simulink model "sst"  (R2025a)
settings: Solver=ode1be  StartTime=0.0  StopTime=simlength  FixedStep=tc  MaxStep=ts_sim
values from neighbouring files (symbols this model uses):
  Adrso = eye(2) + Arso*ts_inv    [design_model.m]
  alpha = 35    [design_model.m]
  C1 = 0.5    [design_model.m]
  Crso = [1 0]    [design_model.m]
  DThs_init = 0    [design_model.m]
  E0 = 3.485    [design_model.m]
  E1 = 0.2156    [design_model.m]
  E2 = 0    [design_model.m]
  E3 = 0    [design_model.m]
  E_1 = -1.031    [design_model.m]
  Elog = -0.05    [design_model.m]
  fPWM_DAB = fPWM_INV    (= 35000)    [design_model.m]
  fPWM_INV = 35e3    (= 35000)    [design_model.m]
  freq = 50    [design_model.m]
  I_FS = Iout_ac_rms_nom * sqrt(2) * margin_factor    [design_model.m]
  ki_i_dab = 18    [design_model.m]
  ki_pll = 3140    [design_model.m]
  ki_v_dab = 45    [design_model.m]
  kp_i_dab = 2    [design_model.m]
  kp_pll = 314    [design_model.m]
  kp_v_dab = 8    [design_model.m]
  Ldrso = acker(Adrso',Crso',polesdrso)'    [design_model.m]
  M = 125    [design_model.m]
  number_of_cells = 30    [design_model.m]
  Q = 1000    [design_model.m]
  q1Kalman = ts_inv^2    (= 8.16326530612e-10)    [design_model.m]
  q2Kalman = ts_inv^1    (= 2.85714285714e-05)    [design_model.m]
  q3Kalman = 0    [design_model.m]
  R0 = 0.0035    [design_model.m]
  R1 = 0.0035    [design_model.m]
  rKalman = 1    [design_model.m]
  Tambient = 40    [design_model.m]
  tc = ts_inv/200    (= 1.42857142857e-07)    [design_model.m]
  ts_afe = ts_inv    (= 2.85714285714e-05)    [design_model.m]
  ts_dab = tPWM_DAB*2    (= 5.71428571429e-05)    [design_model.m]
  ts_inv = tPWM_INV    (= 2.85714285714e-05)    [design_model.m]
  V_FS = Vout_dc_nom * margin_factor    (= 500)    [design_model.m]
  weigth = 0.6/6    (= 0.1)    [design_model.m]
undefined symbols (not defined in the file or in its folder): Aresd, Bresd, Cresd, dead_time_DAB, dead_time_INV, iph_grid_pu_ref, ki_afe, kp_afe, LFu1_AFE, n_modules, omega_grid_nom, RLFu1_AFE, ts_battery, tsample, V_phase_normalization_factor, Vdab2_dc_nom
libraries: fl_lib x280, nesl_utility x188, ee_lib x41, cstblocks x4, single_phase_transformer_lib x2, lithium_ion_cell_lib x1, simulink x1
(part 2 of 12)

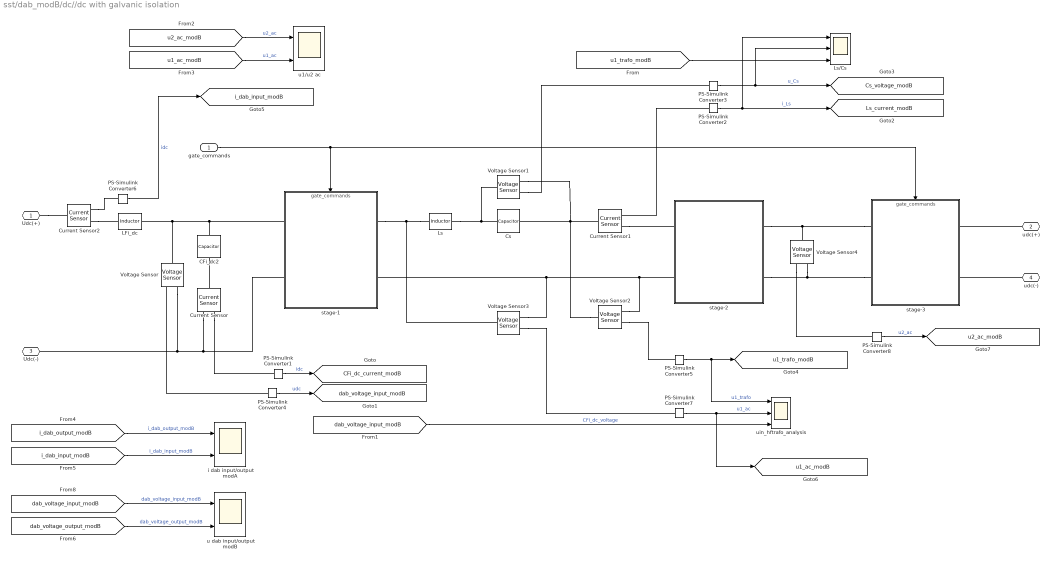
== system sst/dab_modB/dc//dc with galvanic isolation ==
  gate_commands : Inport
  CFi_dc2 : fl_lib/Electrical/Electrical Elements/Capacitor  c=CFi_dc1 F  r=RCFi_dc1_internal Ohm  g=0 1/Ohm  i_specify=off  i_priority=None  i=0 A  i_nominal_specify=off  i_nominal_value=1  i_nominal_unit=A  v_specify=off  v_priority=None  v=0 V  v_nominal_specify=off  v_nominal_value=1  v_nominal_unit=V  vc_specify=off  vc_priority=High  vc=0 V  vc_nominal_specify=off  vc_nominal_value=1  vc_nominal_unit=V
  Cs : fl_lib/Electrical/Electrical Elements/Capacitor  c=Cs1 F  r=1e-6 Ohm  g=0 1/Ohm  i_specify=off  i_priority=None  i=0 A  i_nominal_specify=off  i_nominal_value=1  i_nominal_unit=A  v_specify=off  v_priority=None  v=0 V  v_nominal_specify=off  v_nominal_value=1  v_nominal_unit=V  vc_specify=off  vc_priority=High  vc=0 V  vc_nominal_specify=off  vc_nominal_value=1  vc_nominal_unit=V
  Current Sensor : fl_lib/Electrical/Electrical Sensors/Current Sensor
  Current Sensor1 : fl_lib/Electrical/Electrical Sensors/Current Sensor
  Current Sensor2 : fl_lib/Electrical/Electrical Sensors/Current Sensor
  LFi_dc : fl_lib/Electrical/Electrical Elements/Inductor  l=LFi_dc H  r=RLFi_dc Ohm  g=1e-9 1/Ohm  i_specify=off  i_priority=None  i=0 A  i_nominal_specify=off  i_nominal_value=1  i_nominal_unit=A  v_specify=off  v_priority=None  v=0 V  v_nominal_specify=off  v_nominal_value=1  v_nominal_unit=V  i_L_specify=off  i_L_priority=High  i_L=0 A  i_L_nominal_specify=off  i_L_nominal_value=1  i_L_nominal_unit=A
  Ls : fl_lib/Electrical/Electrical Elements/Inductor  l=Ls1 H  r=0 Ohm  g=1e-9 1/Ohm  i_specify=off  i_priority=None  i=0 A  i_nominal_specify=off  i_nominal_value=1  i_nominal_unit=A  v_specify=off  v_priority=None  v=0 V  v_nominal_specify=off  v_nominal_value=1  v_nominal_unit=V  i_L_specify=off  i_L_priority=High  i_L=0 A  i_L_nominal_specify=off  i_L_nominal_value=1  i_L_nominal_unit=A
  Ls/Cs : Scope  NumInputPorts=3
      settings: SampleTime=tc  ActiveDisplayYMinimum=-8555.3769671330647  ActiveDisplayYMaximum=8509.2940450823044
  PS-Simulink Converter1 : nesl_utility/PS-Simulink Converter  PhysicalDomain=network_engine_domain  SubClassName=ps_output  LeftPortType=input  RightPortType=output  PseudoPeriodic=off  Frequencies=[]  VectorFormat=1-D array  Unit=A  AffineConversion=on
  PS-Simulink Converter2 : nesl_utility/PS-Simulink Converter  PhysicalDomain=network_engine_domain  SubClassName=ps_output  LeftPortType=input  RightPortType=output  PseudoPeriodic=off  Frequencies=[]  VectorFormat=1-D array  Unit=A  AffineConversion=on
  PS-Simulink Converter{3..5,7..8} (5 alike) : nesl_utility/PS-Simulink Converter  PhysicalDomain=network_engine_domain  SubClassName=ps_output  LeftPortType=input  RightPortType=output  PseudoPeriodic=off  Frequencies=[]  VectorFormat=1-D array  Unit=V  AffineConversion=on
  PS-Simulink Converter6 : nesl_utility/PS-Simulink Converter  PhysicalDomain=network_engine_domain  SubClassName=ps_output  LeftPortType=input  RightPortType=output  PseudoPeriodic=off  Frequencies=[]  VectorFormat=1-D array  Unit=A  AffineConversion=on
  Voltage Sensor{,1..4} (5 alike) : fl_lib/Electrical/Electrical Sensors/Voltage Sensor
  i dab input/output modA : Scope  NumInputPorts=2
      settings: SampleTime=tc  ActiveDisplayYMinimum=49.856547808264907  ActiveDisplayYMaximum=125.72881684551226  DataLoggingVariableName=ScopeData9
  stage-1 : Subsystem
      settings: PortSchema="{\"entries\":[{\"content\":{\"sides\":[{\"content\":{\"connectorIds\":[\"LConn1\",\"LConn2\"]},\"type\":\"ConnectorPlacement.EquallySpacedRectSide\",\"uuid\":\"c872503a-61af-4937-bdf2-4de4f8645573\"},{\"content\":{\"connectorIds\":[\"RConn1\",\"RConn2\"],\"side\":\"RIGHT\"},\"type\":\"ConnectorPlacement.EquallySpacedRectSide\",\"uuid\":\"3b83f060-86a2-4569-84b5-d9f7c0485347\"},{\"content\":{\"connectorIds\":[\"In1\"],\"side\":\"TOP\"},\"type\":\"ConnectorPlacement.EquallySpacedRectSide\",\"uuid\":\"bf191d46-ce71-4d15-9dd0-24cc57253577\"}]},\"type\":\"ConnectorPlacement.EquallySpacedConnector\",\"uuid\":\"1b28ceee-25d0-45ae-a3c4-c2563f0d63ba\"}],\"packageUris\":[\"http://schema.mathworks.com/mf0/Connector/R2020b\"],\"version\":\"1.0\"}"
  stage-2 : Subsystem
  stage-3 : Subsystem
      settings: PortSchema="{\"entries\":[{\"content\":{\"sides\":[{\"content\":{\"connectorIds\":[\"LConn1\",\"LConn2\"]},\"type\":\"ConnectorPlacement.EquallySpacedRectSide\",\"uuid\":\"c872503a-61af-4937-bdf2-4de4f8645573\"},{\"content\":{\"connectorIds\":[\"RConn1\",\"RConn2\"],\"side\":\"RIGHT\"},\"type\":\"ConnectorPlacement.EquallySpacedRectSide\",\"uuid\":\"3b83f060-86a2-4569-84b5-d9f7c0485347\"},{\"content\":{\"connectorIds\":[\"In1\"],\"side\":\"TOP\"},\"type\":\"ConnectorPlacement.EquallySpacedRectSide\",\"uuid\":\"bf191d46-ce71-4d15-9dd0-24cc57253577\"}]},\"type\":\"ConnectorPlacement.EquallySpacedConnector\",\"uuid\":\"1b28ceee-25d0-45ae-a3c4-c2563f0d63ba\"}],\"packageUris\":[\"http://schema.mathworks.com/mf0/Connector/R2020b\"],\"version\":\"1.0\"}"
  u dab input/output modB : Scope  NumInputPorts=2
      settings: SampleTime=tc  ActiveDisplayYMinimum=-3745.5802333321844  ActiveDisplayYMaximum=2860.9744612967625  DataLoggingVariableName=ScopeData11
  u1/u2 ac : Scope  NumInputPorts=2
      settings: SampleTime=tc  ActiveDisplayYMinimum=-24024.630641506188  ActiveDisplayYMaximum=24011.441993829012  DataLoggingVariableName=ScopeData5
  uin_hftrafo_analysis : Scope  NumInputPorts=3
      settings: SampleTime=tc  ActiveDisplayYMinimum=-13105.49054417162  ActiveDisplayYMaximum=11952.045335245366
  Udc(+) : PMIOPort  Side=Left
  udc(+) : PMIOPort  Port=2  Side=Right
  Udc(-) : PMIOPort  Port=3  Side=Left
  udc(-) : PMIOPort  Port=4  Side=Right
  tag scope: CFi_dc_current_modB=global, Cs_voltage_modB=global, Ls_current_modB=global, dab_voltage_input_modB=global, i_dab_input_modB=global, u1_ac_modB=global, u1_trafo_modB=global, u2_ac_modB=global
  wires:
  [u1_ac_modB] -> u1/u2 ac/2  "u1_ac"
  [u2_ac_modB] -> u1/u2 ac/1  "u2_ac"
  PS-Simulink Converter8/1 -> [u2_ac_modB]  "u2_ac"
  PS-Simulink Converter6/1 -> [i_dab_input_modB]  "idc"
  [dab_voltage_input_modB] -> uin_hftrafo_analysis/3  "CFi_dc_voltage"
  PS-Simulink Converter7/1 -> uin_hftrafo_analysis/2, [u1_ac_modB]  "u1_ac"
  [u1_trafo_modB] -> Ls/Cs/3
  PS-Simulink Converter5/1 -> [u1_trafo_modB], uin_hftrafo_analysis/1  "u1_trafo"
  PS-Simulink Converter3/1 -> [Cs_voltage_modB], Ls/Cs/2  "u_Cs"
  PS-Simulink Converter2/1 -> [Ls_current_modB], Ls/Cs/1  "i_Ls"
  PS-Simulink Converter4/1 -> [dab_voltage_input_modB]  "udc"
  PS-Simulink Converter1/1 -> [CFi_dc_current_modB]  "idc"
  gate_commands/1 -> stage-1/1(gate_commands), stage-3/1(gate_commands)
  [i_dab_input_modB] -> i dab input/output modA/2  "i_dab_input_modB"
  [i_dab_output_modB] -> i dab input/output modA/1  "i_dab_output_modB"
  [dab_voltage_input_modB] -> u dab input/output modB/1  "dab_voltage_input_modB"
  [dab_voltage_output_modB] -> u dab input/output modB/2  "dab_voltage_output_modB"
  connections:
  Voltage Sensor4/RConn1 -- PS-Simulink Converter8/LConn1
  Current Sensor2/RConn1 -- PS-Simulink Converter6/LConn1
  Udc(+)/RConn1 -- Current Sensor2/LConn1
  Current Sensor2/RConn2 -- LFi_dc/LConn1
  udc(-)/RConn1 -- stage-3/RConn2
  udc(+)/RConn1 -- stage-3/RConn1
  stage-3/LConn2 -- Voltage Sensor4/RConn2 -- stage-2/RConn2
  stage-3/LConn1 -- Voltage Sensor4/LConn1 -- stage-2/RConn1
  Voltage Sensor3/RConn1 -- PS-Simulink Converter7/LConn1
  Voltage Sensor1/LConn1 -- Cs/LConn1 -- Ls/RConn1
  Voltage Sensor2/LConn1 -- Cs/RConn1 -- Current Sensor1/LConn1 -- Voltage Sensor1/RConn2
  Voltage Sensor2/RConn1 -- PS-Simulink Converter5/LConn1
  Voltage Sensor1/RConn1 -- PS-Simulink Converter3/LConn1
  PS-Simulink Converter2/LConn1 -- Current Sensor1/RConn1
  Current Sensor1/RConn2 -- stage-2/LConn1
  Ls/LConn1 -- Voltage Sensor3/LConn1 -- stage-1/LConn1
  PS-Simulink Converter4/LConn1 -- Voltage Sensor/RConn1
  Current Sensor/RConn1 -- PS-Simulink Converter1/LConn1
  Current Sensor/LConn1 -- CFi_dc2/RConn1
  Voltage Sensor/RConn2 -- Udc(-)/RConn1 -- Current Sensor/RConn2 -- stage-1/RConn2
  Voltage Sensor/LConn1 -- LFi_dc/RConn1 -- CFi_dc2/LConn1 -- stage-1/RConn1
  Voltage Sensor3/RConn2 -- stage-1/LConn2 -- Voltage Sensor2/RConn2 -- stage-2/LConn2

== system sst/dab_modB/single_phase_ui_measure1 ==
  Bus Creator : BusCreator  Inputs=2
  Current Sensor : fl_lib/Electrical/Electrical Sensors/Current Sensor
  Selector : Selector  InputPortWidth=2  IndexOptions=Index vector (dialog)  Indices=2  OutputSizes=1
  Selector1 : Selector  InputPortWidth=2  IndexOptions=Index vector (dialog)  Indices=1  OutputSizes=1
  Voltage Sensor : fl_lib/Electrical/Electrical Sensors/Voltage Sensor
  dab input modB : Scope  NumInputPorts=2
      settings: SampleTime=tc  ActiveDisplayYMinimum=-212.36678678828113  ActiveDisplayYMaximum=307.17150645761535  DataLoggingVariableName=ScopeData2
  iph : nesl_utility/PS-Simulink Converter  PhysicalDomain=network_engine_domain  SubClassName=ps_output  LeftPortType=input  RightPortType=output  PseudoPeriodic=off  Frequencies=[]  VectorFormat=1-D array  Unit=A  AffineConversion=off
  uph : nesl_utility/PS-Simulink Converter  PhysicalDomain=network_engine_domain  SubClassName=ps_output  LeftPortType=input  RightPortType=output  PseudoPeriodic=off  Frequencies=[]  VectorFormat=1-D array  Unit=V  AffineConversion=off
  Udc(+) : PMIOPort  Side=Left
  udc(+) : PMIOPort  Port=2  Side=Right
  Udc(-) : PMIOPort  Port=3  Side=Left
  udc(-) : PMIOPort  Port=4  Side=Right
  tag scope: current_battery_modB=global, voltage_battery_modB=global
  wires:
  Selector/1 -> [voltage_battery_modB], dab input modB/2  "voltage_battery"
  Selector1/1 -> dab input modB/1, [current_battery_modB]  "current_battery"
  uph/1 -> Bus Creator/2  "uph"
  iph/1 -> Bus Creator/1  "iph"
  Bus Creator/1 -> Selector1/1, Selector/1  "ui_data"
  connections:
  udc(-)/RConn1 -- Udc(-)/RConn1 -- Voltage Sensor/RConn2
  Voltage Sensor/RConn1 -- uph/LConn1
  Current Sensor/RConn2 -- udc(+)/RConn1
  Udc(+)/RConn1 -- Current Sensor/LConn1 -- Voltage Sensor/LConn1
  iph/LConn1 -- Current Sensor/RConn1

== system sst/dab_modB/ui_measure ==
  Bus Creator : BusCreator  Inputs=2
  Current Sensor : fl_lib/Electrical/Electrical Sensors/Current Sensor
  Selector : Selector  InputPortWidth=2  IndexOptions=Index vector (dialog)  Indices=2  OutputSizes=1
  Selector1 : Selector  InputPortWidth=2  IndexOptions=Index vector (dialog)  Indices=1  OutputSizes=1
  Voltage Sensor : fl_lib/Electrical/Electrical Sensors/Voltage Sensor
  dab output modB : Scope  NumInputPorts=2
      settings: SampleTime=tc  ActiveDisplayYMinimum=-324379.544123381  ActiveDisplayYMaximum=2.4176410117358118E+6  DataLoggingVariableName=ScopeData2
  iph : nesl_utility/PS-Simulink Converter  PhysicalDomain=network_engine_domain  SubClassName=ps_output  LeftPortType=input  RightPortType=output  PseudoPeriodic=off  Frequencies=[]  VectorFormat=1-D array  Unit=A  AffineConversion=off
  uph : nesl_utility/PS-Simulink Converter  PhysicalDomain=network_engine_domain  SubClassName=ps_output  LeftPortType=input  RightPortType=output  PseudoPeriodic=off  Frequencies=[]  VectorFormat=1-D array  Unit=V  AffineConversion=off
  Udc(+) : PMIOPort  Side=Left
  udc(+) : PMIOPort  Port=2  Side=Right
  Udc(-) : PMIOPort  Port=3  Side=Left
  udc(-) : PMIOPort  Port=4  Side=Right
  tag scope: dab_current_output_modB=global, dab_voltage_output_modB=global
  wires:
  uph/1 -> Bus Creator/2  "uph"
  iph/1 -> Bus Creator/1  "iph"
  Bus Creator/1 -> Selector1/1, Selector/1  "ui_data"
  Selector/1 -> [dab_voltage_output_modB]
  Selector1/1 -> [dab_current_output_modB]
  [dab_voltage_output_modB] -> dab output modB/2  "dab_voltage_output_modB"
  [dab_current_output_modB] -> dab output modB/1  "dab_current_output_modB"
  connections:
  udc(-)/RConn1 -- Udc(-)/RConn1 -- Voltage Sensor/RConn2
  Voltage Sensor/RConn1 -- uph/LConn1
  Current Sensor/RConn2 -- udc(+)/RConn1
  Udc(+)/RConn1 -- Current Sensor/LConn1 -- Voltage Sensor/LConn1
  iph/LConn1 -- Current Sensor/RConn1

== system sst/inverter_modA/acquisition_and_scaling_voltage ==
  in : Inport
  1/Ti1 : Gain  Gain=1/V_FS  SaturateOnIntegerOverflow=on  OutDataTypeStr=Inherit: Same as input  ParamDataTypeStr=Inherit: Same as input
  1/Ti2 : Gain  Gain=1/n_modules  SaturateOnIntegerOverflow=on  OutDataTypeStr=Inherit: Same as input  ParamDataTypeStr=Inherit: Same as input
  Unit Delay4 : UnitDelay  SampleTime=ts_inv  HasFrameUpgradeWarning=on
  Zero-Order Hold2 : ZeroOrderHold  SampleTime=ts_inv
  out : Outport
  wires:
  1/Ti1/1 -> Unit Delay4/1
  Zero-Order Hold2/1 -> 1/Ti2/1
  Unit Delay4/1 -> out/1
  in/1 -> Zero-Order Hold2/1
  1/Ti2/1 -> 1/Ti1/1

== system sst/inverter_modA/single phase inverter ==
  gate_commands : Inport
  Current Sensor : fl_lib/Electrical/Electrical Sensors/Current Sensor
  HBridgeIdeal : Subsystem
  HBridgeMosfet : Subsystem  Commented=on
  HBridgeThermal : Subsystem  Commented=on
  Voltage Sensor1 : fl_lib/Electrical/Electrical Sensors/Voltage Sensor
  iph : nesl_utility/PS-Simulink Converter  PhysicalDomain=network_engine_domain  SubClassName=ps_output  LeftPortType=input  RightPortType=output  PseudoPeriodic=off  Frequencies=[]  VectorFormat=1-D array  Unit=A  AffineConversion=off
  uph1 : nesl_utility/PS-Simulink Converter  PhysicalDomain=network_engine_domain  SubClassName=ps_output  LeftPortType=input  RightPortType=output  PseudoPeriodic=off  Frequencies=[]  VectorFormat=1-D array  Unit=V  AffineConversion=off
  uac_out(+) : PMIOPort  Side=Left
  uac_out(-) : PMIOPort  Port=2  Side=Left
  udc(+) : PMIOPort  Port=3  Side=Right
  udc(-) : PMIOPort  Port=4  Side=Right
  tag scope: is_inv_modA=global, us_inv_modA=global
  wires:
  iph/1 -> [is_inv_modA]  "iph"
  uph1/1 -> [us_inv_modA]  "uph"
  gate_commands/1 -> HBridgeIdeal/1(gate_commands)
  connections:
  Current Sensor/RConn1 -- iph/LConn1
  Current Sensor/RConn2 -- Voltage Sensor1/LConn1 -- uac_out(+)/RConn1
  Voltage Sensor1/RConn1 -- uph1/LConn1
  Voltage Sensor1/RConn2 -- HBridgeIdeal/RConn2 -- uac_out(-)/RConn1
  HBridgeIdeal/LConn1 -- udc(+)/RConn1
  HBridgeIdeal/RConn1 -- Current Sensor/LConn1
  HBridgeIdeal/LConn2 -- udc(-)/RConn1

== system sst/inverter_modA/single phase inverter control ==
  Bus Creator : BusCreator  Inputs=4
  Bus Creator1 : BusCreator  Inputs=3
  Bus Creator2 : BusCreator  Inputs=2
  acquisition_and_scaling_current : Subsystem
  pwm : Subsystem
  references_generator_modA : Subsystem
  rpi_based_single_phase_inverter_ctrl : Subsystem
  single phase inverter tracking current : Scope  NumInputPorts=2
      settings: SampleTime=tc  ActiveDisplayYMinimum=-2.0191055995291  ActiveDisplayYMaximum=2.2692364997570564  DataLoggingVariableName=ScopeData3
  gate_commands : Outport
  wires:
  pwm/3(m2_top) -> Bus Creator/3
  Bus Creator/1 -> gate_commands/1
  pwm/1(m1_top) -> Bus Creator/1
  pwm/2(m1_bottom) -> Bus Creator/2
  pwm/4(m2_bottom) -> Bus Creator/4
  [is_inv_modA] -> acquisition_and_scaling_current/1(in)
  acquisition_and_scaling_current/1(out) -> rpi_based_single_phase_inverter_ctrl/1(i_out_inverter_pu)  "is_pu"
  rpi_based_single_phase_inverter_ctrl/1(u_ctrl_out) -> pwm/1(vout)
  references_generator_modA/1(i_out_inverter_reference_pu) -> rpi_based_single_phase_inverter_ctrl/2(i_out_inverter_reference_pu)  "is_ref_pu"
  Bus Creator1/1 -> single phase inverter tracking current/2  "is_tracking"
  [is_inv_modA] -> Bus Creator2/2  "is"
  Bus Creator2/1 -> single phase inverter tracking current/1  "load"
  [inverter_voltage_output_modA] -> Bus Creator2/1  "u_out"
  [i_out_inverter_pu_ref_modA] -> Bus Creator1/2  "i_out_inverter_pu_ref"
  [i_out_inverter_pu_modA] -> Bus Creator1/3  "i_out_inverter_pu"
  [id_inv_pu_ref_modA] -> Bus Creator1/1  "id_inv_pu_ref"

== system sst/inverter_modA/single_phase_pll ==
  uin : Inport
  Constant : Constant  Value=2*pi*freq
  Constant2 : Constant  Value=0
  Sum : Sum  Inputs=|++
  Sum1 : Sum  Inputs=|++
  Terminator1 : Terminator
  Terminator2 : Terminator
  Terminator3 : Terminator
  Unit Delay1 : UnitDelay  SampleTime=ts_inv  HasFrameUpgradeWarning=on
  alphabeta2xieta : MATLAB Function  TreatAsAtomicUnit=on  SystemSampleTime=ts_inv
  double_integrator_observer : Subsystem
  freq_pll : Gain  Gain=1/2/pi
  omega_int_ts : Gain  Gain=ts_inv
  pi-ctrl : Subsystem  mask{kp=kp_pll, ki=ki_pll, ts=ts_inv, sat_pos=inf, sat_neg=-inf}
  theta_pll_hat : Gain
  ualpha_pll : Gain
  ubeta_pll : Gain
  ueta_pll : Gain  Gain=-1
  ueta_pll_flt : cstblocks/LTI System  sys=Hd  IC=[]  PadeOrder=0
  uxi_pll : Gain
  uxi_pll_flt : cstblocks/LTI System  sys=Hd  IC=[]  PadeOrder=0
  xieta2alphabeta : MATLAB Function  TreatAsAtomicUnit=on  SystemSampleTime=ts_inv
  Out1 : Outport
  wires:
  Sum/1 -> double_integrator_observer/1(theta), xieta2alphabeta/3(gamma), alphabeta2xieta/3(gamma), Unit Delay1/1
  Unit Delay1/1 -> Sum/2
  alphabeta2xieta/1(xi) -> uxi_pll_flt/1, uxi_pll/1
  xieta2alphabeta/2(beta) -> ubeta_pll/1
  alphabeta2xieta/2(eta) -> ueta_pll_flt/1, ueta_pll/1
  omega_int_ts/1 -> Sum/1
  double_integrator_observer/1(theta_hat) -> theta_pll_hat/1  "theta_hat"
  uin/1 -> alphabeta2xieta/1(alpha)
  freq_pll/1 -> Terminator1/1  "freq_pll"
  ueta_pll_flt/1 -> xieta2alphabeta/2(eta)
  uxi_pll_flt/1 -> xieta2alphabeta/1(xi)
  ueta_pll/1 -> pi-ctrl/1(x)
  Sum1/1 -> freq_pll/1, omega_int_ts/1  "freq_pll"
  Constant2/1 -> pi-ctrl/2(xref)
  uxi_pll/1 -> Terminator2/1
  ubeta_pll/1 -> alphabeta2xieta/2(beta)
  xieta2alphabeta/1(alpha) -> ualpha_pll/1
  ualpha_pll/1 -> Terminator3/1
  pi-ctrl/1(u) -> Sum1/1
  Constant/1 -> Sum1/2
  theta_pll_hat/1 -> Out1/1  "theta_pll_hat"

== system sst/inverter_modB/acquisition_and_scaling_voltage ==
  in : Inport
  1/Ti1 : Gain  Gain=1/V_FS  SaturateOnIntegerOverflow=on  OutDataTypeStr=Inherit: Same as input  ParamDataTypeStr=Inherit: Same as input
  1/Ti2 : Gain  Gain=1/n_modules  SaturateOnIntegerOverflow=on  OutDataTypeStr=Inherit: Same as input  ParamDataTypeStr=Inherit: Same as input
  Unit Delay4 : UnitDelay  SampleTime=ts_inv  HasFrameUpgradeWarning=on
  Zero-Order Hold2 : ZeroOrderHold  SampleTime=ts_inv
  out : Outport
  wires:
  in/1 -> Zero-Order Hold2/1
  Unit Delay4/1 -> out/1
  Zero-Order Hold2/1 -> 1/Ti2/1
  1/Ti1/1 -> Unit Delay4/1
  1/Ti2/1 -> 1/Ti1/1

== system sst/inverter_modB/single phase inverter ==
  gate_commands : Inport
  Current Sensor : fl_lib/Electrical/Electrical Sensors/Current Sensor
  HBridgeIdeal : Subsystem
  HBridgeMosfet : Subsystem  Commented=on
  HBridgeThermal : Subsystem  Commented=on
  Voltage Sensor1 : fl_lib/Electrical/Electrical Sensors/Voltage Sensor
  iph : nesl_utility/PS-Simulink Converter  PhysicalDomain=network_engine_domain  SubClassName=ps_output  LeftPortType=input  RightPortType=output  PseudoPeriodic=off  Frequencies=[]  VectorFormat=1-D array  Unit=A  AffineConversion=off
  uph1 : nesl_utility/PS-Simulink Converter  PhysicalDomain=network_engine_domain  SubClassName=ps_output  LeftPortType=input  RightPortType=output  PseudoPeriodic=off  Frequencies=[]  VectorFormat=1-D array  Unit=V  AffineConversion=off
  uac_out(+) : PMIOPort  Side=Left
  uac_out(-) : PMIOPort  Port=2  Side=Left
  udc(+) : PMIOPort  Port=3  Side=Right
  udc(-) : PMIOPort  Port=4  Side=Right
  tag scope: is_inv_modB=global, us_inv_modB=global
  wires:
  gate_commands/1 -> HBridgeIdeal/1(gate_commands)
  uph1/1 -> [us_inv_modB]  "uph"
  iph/1 -> [is_inv_modB]  "iph"
  connections:
  HBridgeIdeal/LConn2 -- udc(-)/RConn1
  HBridgeIdeal/RConn1 -- Current Sensor/LConn1
  HBridgeIdeal/LConn1 -- udc(+)/RConn1
  uac_out(-)/RConn1 -- HBridgeIdeal/RConn2 -- Voltage Sensor1/RConn2
  Voltage Sensor1/RConn1 -- uph1/LConn1
  uac_out(+)/RConn1 -- Voltage Sensor1/LConn1 -- Current Sensor/RConn2
  Current Sensor/RConn1 -- iph/LConn1

== system sst/inverter_modB/single phase inverter control ==
  Bus Creator : BusCreator  Inputs=4
  Bus Creator1 : BusCreator  Inputs=3
  Bus Creator2 : BusCreator  Inputs=2
  acquisition_and_scaling_current : Subsystem
  pwm : Subsystem
  references_generator_modB : Subsystem
  rpi_based_single_phase_inverter_ctrl : Subsystem
  single phase inverter tracking current : Scope  NumInputPorts=2
      settings: SampleTime=tc  ActiveDisplayYMinimum=-9.23533057586284  ActiveDisplayYMaximum=5.8557270929450596  DataLoggingVariableName=ScopeData3
  gate_commands : Outport
  wires:
  [id_inv_pu_ref_modB] -> Bus Creator1/1  "id_inv_pu_ref"
  [i_out_inverter_pu_modB] -> Bus Creator1/3  "i_out_inverter_pu"
  [i_out_inverter_pu_ref_modB] -> Bus Creator1/2  "i_out_inverter_pu_ref"
  [inverter_voltage_output_modB] -> Bus Creator2/1  "u_out"
  Bus Creator2/1 -> single phase inverter tracking current/1  "load"
  [is_inv_modB] -> Bus Creator2/2  "is"
  Bus Creator1/1 -> single phase inverter tracking current/2  "is_tracking"
  references_generator_modB/1(i_out_inverter_reference_pu) -> rpi_based_single_phase_inverter_ctrl/2(i_out_inverter_reference_pu)  "is_ref_pu"
  rpi_based_single_phase_inverter_ctrl/1(u_ctrl_out) -> pwm/1(vout)
  acquisition_and_scaling_current/1(out) -> rpi_based_single_phase_inverter_ctrl/1(i_out_inverter_pu)  "is_pu"
  [is_inv_modB] -> acquisition_and_scaling_current/1(in)
  pwm/4(m2_bottom) -> Bus Creator/4
  pwm/2(m1_bottom) -> Bus Creator/2
  pwm/1(m1_top) -> Bus Creator/1
  Bus Creator/1 -> gate_commands/1
  pwm/3(m2_top) -> Bus Creator/3

== system sst/inverter_modB/single_phase_pll ==
  uin : Inport
  Constant : Constant  Value=2*pi*freq
  Constant2 : Constant  Value=0
  Sum : Sum  Inputs=|++
  Sum1 : Sum  Inputs=|++
  Terminator1 : Terminator
  Terminator2 : Terminator
  Terminator3 : Terminator
  Unit Delay1 : UnitDelay  SampleTime=ts_inv  HasFrameUpgradeWarning=on
  alphabeta2xieta : MATLAB Function  TreatAsAtomicUnit=on  SystemSampleTime=ts_inv
  double_integrator_observer : Subsystem
  freq_pll : Gain  Gain=1/2/pi
  omega_int_ts : Gain  Gain=ts_inv
  pi-ctrl : Subsystem  mask{kp=kp_pll, ki=ki_pll, ts=ts_inv, sat_pos=inf, sat_neg=-inf}
  theta_pll_hat : Gain
  ualpha_pll : Gain
  ubeta_pll : Gain
  ueta_pll : Gain  Gain=-1
  ueta_pll_flt : cstblocks/LTI System  sys=Hd  IC=[]  PadeOrder=0
  uxi_pll : Gain
  uxi_pll_flt : cstblocks/LTI System  sys=Hd  IC=[]  PadeOrder=0
  xieta2alphabeta : MATLAB Function  TreatAsAtomicUnit=on  SystemSampleTime=ts_inv
  phase_pll_hat : Outport
  wires:
  theta_pll_hat/1 -> phase_pll_hat/1  "theta_pll_hat"
  Constant/1 -> Sum1/2
  pi-ctrl/1(u) -> Sum1/1
  ualpha_pll/1 -> Terminator3/1
  xieta2alphabeta/1(alpha) -> ualpha_pll/1
  ubeta_pll/1 -> alphabeta2xieta/2(beta)
  uxi_pll/1 -> Terminator2/1
  Constant2/1 -> pi-ctrl/2(xref)
  Sum1/1 -> omega_int_ts/1, freq_pll/1  "freq_pll"
  ueta_pll/1 -> pi-ctrl/1(x)
  uxi_pll_flt/1 -> xieta2alphabeta/1(xi)
  ueta_pll_flt/1 -> xieta2alphabeta/2(eta)
  freq_pll/1 -> Terminator1/1  "freq_pll"
  uin/1 -> alphabeta2xieta/1(alpha)
  double_integrator_observer/1(theta_hat) -> theta_pll_hat/1  "theta_hat"
  omega_int_ts/1 -> Sum/1
  alphabeta2xieta/2(eta) -> ueta_pll/1, ueta_pll_flt/1
  xieta2alphabeta/2(beta) -> ubeta_pll/1
  alphabeta2xieta/1(xi) -> uxi_pll/1, uxi_pll_flt/1
  Unit Delay1/1 -> Sum/2
  Sum/1 -> Unit Delay1/1, alphabeta2xieta/3(gamma), xieta2alphabeta/3(gamma), double_integrator_observer/1(theta)

== system sst/line_source/phase_gen ==
  Constant4 : Constant  Value=omega_grid_nom
  Sum4 : Sum  SaturateOnIntegerOverflow=on
  Unit Delay1 : UnitDelay  SampleTime=ts_afe  HasFrameUpgradeWarning=on
  bounder1 : MATLAB Function  TreatAsAtomicUnit=on  SystemSampleTime=ts_inv
  kp2 : Gain  Gain=ts_afe  SaturateOnIntegerOverflow=on  OutDataTypeStr=Inherit: Same as input  ParamDataTypeStr=Inherit: Same as input
  phase_gen : Outport  VectorParamsAs1DForOutWhenUnconnected=off
  wires:
  bounder1/1(y) -> Unit Delay1/1  "grid_emu_phase"
  kp2/1 -> Sum4/1
  Constant4/1 -> kp2/1
  Unit Delay1/1 -> Sum4/2, phase_gen/1
  Sum4/1 -> bounder1/1(u)

== system sst/battery/LithiumIonBattery/SOC_estimator ==
  Kalman_observer : Subsystem
  SOC*/SOC : Scope  NumInputPorts=2
      settings: SampleTime=ts_battery  ActiveDisplayYMinimum=-0.16149  ActiveDisplayYMaximum=0.90685
  Selector1 : Selector  InputPortWidth=3  IndexOptions=Index vector (dialog)  Indices=3  OutputSizes=1
  h_hat/h : Scope  NumInputPorts=2
      settings: SampleTime=ts_battery  ActiveDisplayYMinimum=-0.13002  ActiveDisplayYMaximum=0.15534  DataLoggingVariableName=ScopeData2
  i_out/v_out : Scope  NumInputPorts=2
      settings: SampleTime=ts_battery  ActiveDisplayYMinimum=-467.64425  ActiveDisplayYMaximum=280.87629  DataLoggingVariableName=ScopeData3
  soc/iout : Scope  NumInputPorts=2
      settings: SampleTime=ts_battery  ActiveDisplayYMinimum=0.19925  ActiveDisplayYMaximum=0.20008  DataLoggingVariableName=ScopeData4
  wires:
  Kalman_observer/2(SOC) -> SOC*/SOC/2
  Kalman_observer/1(x(k+1|k)) -> Selector1/1
  [im] -> i_out/v_out/1  "im+noise"
  [h] -> h_hat/h/2
  [SOC] -> soc/iout/1, SOC*/SOC/1
  Selector1/1 -> h_hat/h/1  "h_hat(z)"
  [vout] -> Kalman_observer/1(vout(k)), i_out/v_out/2
  [icell] -> soc/iout/2

== system sst/battery/LithiumIonBattery/lithium ion cell analytical ocv ==
  Current Sensor : fl_lib/Electrical/Electrical Sensors/Current Sensor
  Electrical Reference : fl_lib/Electrical/Electrical Elements/Electrical Reference
  PS Constant : fl_lib/Physical Signals/Sources/PS Constant  constant=298.15 K
  PS-Simulink Converter{,1..4} (5 alike) : nesl_utility/PS-Simulink Converter  PhysicalDomain=network_engine_domain  SubClassName=ps_output  LeftPortType=input  RightPortType=output  PseudoPeriodic=off  Frequencies=[]  VectorFormat=1-D array  Unit=inherit  AffineConversion=off
  Voltage Sensor : fl_lib/Electrical/Electrical Sensors/Voltage Sensor
  lithium-ion battery with analytical OCV : lithium_ion_cell_lib/lithium-ion Cell with analytical OCV  Qcell=Q hr*A  N=number_of_cells  E_1=E1 V  E0=E0 V  E1=E1 V  E2=E2 V  E3=E3 V  Elog=Elog V  R0=R0 Ohm  R1=R1 Ohm  C1=C1 F  M=M V  alpha=alpha  u_specify=off  u_priority=High  u=Vdc V  u_nominal_specify=off  u_nominal_unit=V  u_nominal_value=1  u_ocv_specify=off  u_ocv_priority=High  u_ocv=Vdc V  u_ocv_nominal_specify=off  u_ocv_nominal_unit=V  u_ocv_nominal_value=1  icell_specify=off  icell_priority=None  icell=0 A  icell_nominal_specify=off  icell_nominal_unit=A  icell_nominal_value=1  i_r1_specify=off  i_r1_priority=None  i_r1=0 A  i_r1_nominal_specify=off  i_r1_nominal_unit=A  i_r1_nominal_value=1  z_specify=on  z_priority=High  z=soc_init  z_nominal_specify=off  z_nominal_unit=1  z_nominal_value=1  h_specify=off  h_priority=High  h=0  h_nominal_specify=off  h_nominal_unit=1  h_nominal_value=1
      settings: InternalSimscapePortConfiguration="{\"Bottom\":[],\"Left\":[{\"id\":\"T\",\"label\":\"T\",\"type\":\"input\"}],\"Right\":[{\"id\":\"u_p\",\"label\":\"u+\",\"type\":\"foundation.electrical.electrical\"},{\"id\":\"u_n\",\"label\":\"u-\",\"type\":\"foundation.electrical.electrical\"},{\"id\":\"z_out\",\"label\":\"SOC\",\"type\":\"output\"},{\"id\":\"i_r1_out\",\"label\":\"i_r1\",\"type\":\"output\"},{\"id\":\"h_out\",\"label\":\"hysteresis\",\"type\":\"output\"}],\"Top\":[]}"
  white_noise : Subsystem
  U+ : PMIOPort  Side=Right
  U- : PMIOPort  Port=2  Side=Right
  tag scope: SOC=global, h=global, icell=global, im=global, vout=global
  wires:
  PS-Simulink Converter/1 -> [vout]  "vout(k)"
  PS-Simulink Converter1/1 -> white_noise/1(in)  "i(k)"
  white_noise/1(out) -> [im]
  PS-Simulink Converter4/1 -> [h]  "h(t)"
  PS-Simulink Converter2/1 -> [icell]  "icell"
  PS-Simulink Converter3/1 -> [SOC]  "SOC*"
  connections:
  lithium-ion battery with analytical OCV/LConn1 -- PS Constant/RConn1
  PS-Simulink Converter/LConn1 -- Voltage Sensor/RConn1
  Current Sensor/RConn2 -- Voltage Sensor/LConn1 -- U+/RConn1
  Electrical Reference/LConn1 -- Voltage Sensor/RConn2 -- U-/RConn1 -- lithium-ion battery with analytical OCV/RConn2
  Current Sensor/RConn1 -- PS-Simulink Converter1/LConn1
  lithium-ion battery with analytical OCV/RConn1 -- Current Sensor/LConn1
  lithium-ion battery with analytical OCV/RConn3 -- PS-Simulink Converter3/LConn1
  lithium-ion battery with analytical OCV/RConn4 -- PS-Simulink Converter2/LConn1
  lithium-ion battery with analytical OCV/RConn5 -- PS-Simulink Converter4/LConn1

== system sst/dab_modA/dab_ctrl/modulator1 ==
  phase_displacement : Inport
  Constant : Constant  Value=0.5
  Constant1 : Constant  Value=0
  Constant2 : Constant  Value=-1
  Constant3 : Constant  Value=0.5
  Constant4 : Constant  Value=pi
  Constant5 : Constant  Value=-1
  Constant6 : Constant  Value=pi
  Gain : Gain  Gain=pi/4  OutDataTypeStr=double
  PWM generator 1 : Subsystem  mask{f=fPWM_DAB, m_up=1, m_low=0, dead_time=dead_time_DAB, pos_cmd_gate=15, neg_cmd_gate=-10, polarity=1}
      mask prompts: f "Frequency (Hz)"; m_up "Max Input Modulation Value"; m_low "Min Input Modulation Value"; dead_time "Dead Time (s)"; pos_cmd_gate "Positive Gate Voltage (V)"; neg_cmd_gate "Negative Gate Voltage (V)"; polarity "Polarity (pu)"
  PWM generator 2 : Subsystem  mask{f=fPWM_DAB, m_up=1, m_low=0, dead_time=dead_time_DAB, pos_cmd_gate=15, neg_cmd_gate=-10, polarity=1}
      mask prompts: f "Frequency (Hz)"; m_up "Max Input Modulation Value"; m_low "Min Input Modulation Value"; dead_time "Dead Time (s)"; pos_cmd_gate "Positive Gate Voltage (V)"; neg_cmd_gate "Negative Gate Voltage (V)"; polarity "Polarity (pu)"
  PWM generator 3 : Subsystem  mask{f=fPWM_DAB, m_up=1, m_low=0, dead_time=dead_time_DAB, pos_cmd_gate=15, neg_cmd_gate=-10, polarity=1}
      mask prompts: f "Frequency (Hz)"; m_up "Max Input Modulation Value"; m_low "Min Input Modulation Value"; dead_time "Dead Time (s)"; pos_cmd_gate "Positive Gate Voltage (V)"; neg_cmd_gate "Negative Gate Voltage (V)"; polarity "Polarity (pu)"
  PWM generator 4 : Subsystem  mask{f=fPWM_DAB, m_up=1, m_low=0, dead_time=dead_time_DAB, pos_cmd_gate=15, neg_cmd_gate=-10, polarity=1}
      mask prompts: f "Frequency (Hz)"; m_up "Max Input Modulation Value"; m_low "Min Input Modulation Value"; dead_time "Dead Time (s)"; pos_cmd_gate "Positive Gate Voltage (V)"; neg_cmd_gate "Negative Gate Voltage (V)"; polarity "Polarity (pu)"
  Sum : Sum  Inputs=|++
  dab_modulation : Scope  NumInputPorts=4
      settings: SampleTime=tc  ActiveDisplayYMinimum=-13.125  ActiveDisplayYMaximum=18.125
  gate_Q1 : Outport
  gate_Q2 : Outport  Port=2
  gate_Q3 : Outport  Port=3
  gate_Q4 : Outport  Port=4
  gate_Q5 : Outport  Port=5
  gate_Q6 : Outport  Port=6
  gate_Q7 : Outport  Port=7
  gate_Q8 : Outport  Port=8
  wires:
  PWM generator 2/2(m2) -> gate_Q4/1  "gate_Q4"
  PWM generator 2/1(m1) -> dab_modulation/2, gate_Q3/1  "gate_Q3"
  PWM generator 1/2(m2) -> gate_Q2/1  "gate_Q2"
  PWM generator 1/1(m1) -> gate_Q1/1, dab_modulation/1  "gate_Q1"
  phase_displacement/1 -> Gain/1
  Constant/1 -> PWM generator 2/1(m_index), PWM generator 1/1(m_index)
  Constant1/1 -> PWM generator 1/2(phase)
  Constant2/1 -> PWM generator 2/3(polarity_input), PWM generator 1/3(polarity_input)
  Constant5/1 -> PWM generator 3/3(polarity_input), PWM generator 4/3(polarity_input)
  Gain/1 -> Sum/1, PWM generator 3/2(phase)
  Constant3/1 -> PWM generator 3/1(m_index), PWM generator 4/1(m_index)
  Sum/1 -> PWM generator 4/2(phase)
  PWM generator 3/1(m1) -> gate_Q5/1, dab_modulation/3  "gate_Q5"
  PWM generator 3/2(m2) -> gate_Q6/1  "gate_Q6"
  PWM generator 4/1(m1) -> dab_modulation/4, gate_Q7/1  "gate_Q7"
  PWM generator 4/2(m2) -> gate_Q8/1  "gate_Q8"
  Constant6/1 -> PWM generator 2/2(phase)
  Constant4/1 -> Sum/2

== system sst/dab_modA/dab_ctrl/references ==
  Rate Limiter : RateLimiter  RisingSlewLimit=Vdab2_dc_nom*10  FallingSlewLimit=-Vdab2_dc_nom*10  SampleTimeMode=inherited
  Vout_dc_nom : Step  Time=1e-3  After=Vdab2_dc_nom  SampleTime=0
  vout_ref : Outport
  wires:
  Rate Limiter/1 -> vout_ref/1
  Vout_dc_nom/1 -> Rate Limiter/1

== system sst/dab_modA/dab_ctrl/sampling_i_filter1 ==
  in : Inport
  1/Ti3 : Gain  Gain=1/I_FS  OutDataTypeStr=double  SaturateOnIntegerOverflow=on  ParamDataTypeStr=Inherit: Same as input
  Unit Delay1 : UnitDelay  SampleTime=ts_dab  HasFrameUpgradeWarning=on
  Zero-Order Hold2 : ZeroOrderHold  SampleTime=ts_dab
  out_pu : Outport
  wires:
  in/1 -> 1/Ti3/1
  1/Ti3/1 -> Zero-Order Hold2/1
  Zero-Order Hold2/1 -> Unit Delay1/1
  Unit Delay1/1 -> out_pu/1

== system sst/dab_modA/dab_ctrl/sampling_v_filter1 ==
  in : Inport
  1/Ti3 : Gain  Gain=1/V_FS  OutDataTypeStr=double  SaturateOnIntegerOverflow=on  ParamDataTypeStr=Inherit: Same as input
  Unit Delay1 : UnitDelay  SampleTime=ts_dab  HasFrameUpgradeWarning=on
  Zero-Order Hold2 : ZeroOrderHold  SampleTime=ts_dab
  out_pu : Outport
  wires:
  Zero-Order Hold2/1 -> Unit Delay1/1
  in/1 -> 1/Ti3/1
  1/Ti3/1 -> Zero-Order Hold2/1
  Unit Delay1/1 -> out_pu/1

== system sst/dab_modA/dab_ctrl/sampling_v_filter2 ==
  in : Inport
  1/Ti3 : Gain  Gain=1/V_FS  OutDataTypeStr=double  SaturateOnIntegerOverflow=on  ParamDataTypeStr=Inherit: Same as input
  Saturation : Saturate  UpperLimit=1  LowerLimit=0  OutDataTypeStr=double
  Unit Delay1 : UnitDelay  SampleTime=ts_dab  HasFrameUpgradeWarning=on
  Zero-Order Hold2 : ZeroOrderHold  SampleTime=ts_dab
  out_pu : Outport
  wires:
  in/1 -> 1/Ti3/1
  1/Ti3/1 -> Saturation/1
  Zero-Order Hold2/1 -> Unit Delay1/1
  Saturation/1 -> Zero-Order Hold2/1
  Unit Delay1/1 -> out_pu/1

== system sst/dab_modA/dab_ctrl/vi ctrl ==
  i_dab_input : Inport
  u_dab_output : Inport  Port=2
  u_dab_output_ref : Inport  Port=3
  Bus Creator : BusCreator  Inputs=2
  Bus Creator1 : BusCreator  Inputs=2
  Iout Ctrl : Subsystem
  Vout Ctrl : Subsystem
  dab-tracking : Scope  NumInputPorts=2
      settings: ActiveDisplayYMinimum=-2  ActiveDisplayYMaximum=2  DataLoggingVariableName=ScopeData7
  u_ctrl_out_dab/i_ctrl_out_dab : Scope  NumInputPorts=2
      settings: ActiveDisplayYMinimum=-0.75125269086331614  ActiveDisplayYMaximum=0.35986759850292721
  phase_displacement : Outport
  tag scope: i_ctrl_out_dab=global, i_in_pu_dab=global, u_ctrl_out_dab=global, uout_pu_dab=global, uout_ref_pu_dab=global
  wires:
  i_dab_input/1 -> [i_in_pu_dab], Iout Ctrl/2(iout)
  u_dab_output_ref/1 -> Vout Ctrl/1(vout_ref), [uout_ref_pu_dab]
  u_dab_output/1 -> [uout_pu_dab], Vout Ctrl/2(vout)
  Vout Ctrl/1(ctrlv_out) -> Iout Ctrl/1(iout_ref), [u_ctrl_out_dab]
  Iout Ctrl/1(ctrli_out) -> [i_ctrl_out_dab], phase_displacement/1
  [u_ctrl_out_dab] -> u_ctrl_out_dab/i_ctrl_out_dab/1  "u_ctrl_out_dab"
  [i_ctrl_out_dab] -> u_ctrl_out_dab/i_ctrl_out_dab/2  "i_ctrl_out_dab"
  [i_in_pu_dab] -> Bus Creator1/2  "i_in_pu_dab"
  [u_ctrl_out_dab] -> Bus Creator1/1  "u_ctrl_out_dab"
  [uout_ref_pu_dab] -> Bus Creator/1  "uout_ref_pu_dab"
  [uout_pu_dab] -> Bus Creator/2  "uout_pu_dab"
  Bus Creator/1 -> dab-tracking/1
  Bus Creator1/1 -> dab-tracking/2

== system sst/dab_modA/dc//dc with galvanic isolation/stage-1 ==
  gate_commands : Inport
  Current Sensor : fl_lib/Electrical/Electrical Sensors/Current Sensor
  PS-Simulink Converter1 : nesl_utility/PS-Simulink Converter  PhysicalDomain=network_engine_domain  SubClassName=ps_output  LeftPortType=input  RightPortType=output  PseudoPeriodic=off  Frequencies=[]  VectorFormat=1-D array  Unit=A  AffineConversion=on
  h-bridge_thermal : Subsystem  Commented=on
  h-ideal : Subsystem  Commented=on
  h-mosfet : Subsystem
  uac_1(+) : PMIOPort  Side=Left
  uac_1(-) : PMIOPort  Port=2  Side=Left
  Udc(+) : PMIOPort  Port=3  Side=Right
  Udc(-) : PMIOPort  Port=4  Side=Right
  tag scope: dc_bus_terminal_current_inverter=global
  wires:
  gate_commands/1 -> h-mosfet/1(gate_commands)
  PS-Simulink Converter1/1 -> [dc_bus_terminal_current_inverter]  "idc"
  connections:
  h-mosfet/LConn1 -- uac_1(+)/RConn1
  h-mosfet/LConn2 -- uac_1(-)/RConn1
  h-mosfet/RConn2 -- Udc(-)/RConn1
  Current Sensor/LConn1 -- Udc(+)/RConn1
  h-mosfet/RConn1 -- Current Sensor/RConn2
  PS-Simulink Converter1/LConn1 -- Current Sensor/RConn1

== system sst/dab_modA/dc//dc with galvanic isolation/stage-2 ==
  Current Sensor1 : fl_lib/Electrical/Electrical Sensors/Current Sensor
  PS-Simulink Converter2 : nesl_utility/PS-Simulink Converter  PhysicalDomain=network_engine_domain  SubClassName=ps_output  LeftPortType=input  RightPortType=output  PseudoPeriodic=off  Frequencies=[]  VectorFormat=1-D array  Unit=A  AffineConversion=on
  hf_trafo_center_tap_ss : Subsystem
  uac_1(+) : PMIOPort  Side=Left
  uac_2(+) : PMIOPort  Port=2  Side=Right
  uac_1(-) : PMIOPort  Port=3  Side=Left
  uac_2(-) : PMIOPort  Port=4  Side=Right
  connections:
  Current Sensor1/RConn2 -- uac_2(+)/RConn1
  PS-Simulink Converter2/LConn1 -- Current Sensor1/RConn1
  hf_trafo_center_tap_ss/LConn1 -- uac_1(+)/RConn1
  hf_trafo_center_tap_ss/RConn1 -- Current Sensor1/LConn1
  hf_trafo_center_tap_ss/LConn2 -- uac_1(-)/RConn1
  hf_trafo_center_tap_ss/RConn2 -- uac_2(-)/RConn1

== system sst/dab_modA/dc//dc with galvanic isolation/stage-3 ==
  gate_commands : Inport
  CFi_dc2 : fl_lib/Electrical/Electrical Elements/Capacitor  c=CFi_dc2 F  r=RCFi_dc2_internal Ohm  g=0 1/Ohm  i_specify=off  i_priority=None  i=0 A  i_nominal_specify=off  i_nominal_value=1  i_nominal_unit=A  v_specify=off  v_priority=None  v=0 V  v_nominal_specify=off  v_nominal_value=1  v_nominal_unit=V  vc_specify=off  vc_priority=High  vc=0 V  vc_nominal_specify=off  vc_nominal_value=1  vc_nominal_unit=V
  Current Sensor : fl_lib/Electrical/Electrical Sensors/Current Sensor
  Current Sensor2 : fl_lib/Electrical/Electrical Sensors/Current Sensor
  PS-Simulink Converter1 : nesl_utility/PS-Simulink Converter  PhysicalDomain=network_engine_domain  SubClassName=ps_output  LeftPortType=input  RightPortType=output  PseudoPeriodic=off  Frequencies=[]  VectorFormat=1-D array  Unit=A  AffineConversion=on
  PS-Simulink Converter6 : nesl_utility/PS-Simulink Converter  PhysicalDomain=network_engine_domain  SubClassName=ps_output  LeftPortType=input  RightPortType=output  PseudoPeriodic=off  Frequencies=[]  VectorFormat=1-D array  Unit=A  AffineConversion=on
  h-mosfet : Subsystem
  uac_1(+) : PMIOPort  Side=Left
  uac_1(-) : PMIOPort  Port=2  Side=Left
  udc(+) : PMIOPort  Port=3  Side=Right
  udc(-) : PMIOPort  Port=4  Side=Right
  tag scope: CFi_dc2_current_modA=global, i_dab_output_modA=global
  wires:
  gate_commands/1 -> h-mosfet/1(gate_commands)
  PS-Simulink Converter6/1 -> [CFi_dc2_current_modA]  "i_Ls"
  PS-Simulink Converter1/1 -> [i_dab_output_modA]  "idc"
  connections:
  h-mosfet/RConn1 -- Current Sensor/LConn1 -- CFi_dc2/LConn1
  udc(+)/RConn1 -- Current Sensor/RConn2
  h-mosfet/RConn2 -- Current Sensor2/RConn2 -- udc(-)/RConn1
  h-mosfet/LConn2 -- uac_1(-)/RConn1
  h-mosfet/LConn1 -- uac_1(+)/RConn1
  PS-Simulink Converter6/LConn1 -- Current Sensor2/RConn1
  CFi_dc2/RConn1 -- Current Sensor2/LConn1
  Current Sensor/RConn1 -- PS-Simulink Converter1/LConn1

== system sst/dab_modB/dab_ctrl/modulator1 ==
  phase_displacement : Inport
  Constant : Constant  Value=0.5
  Constant1 : Constant  Value=0
  Constant2 : Constant  Value=-1
  Constant3 : Constant  Value=0.5
  Constant4 : Constant  Value=pi
  Constant5 : Constant  Value=-1
  Constant6 : Constant  Value=pi
  Gain : Gain  Gain=pi/4  OutDataTypeStr=double
  PWM generator 1 : Subsystem  mask{f=fPWM_DAB, m_up=1, m_low=0, dead_time=dead_time_DAB, pos_cmd_gate=15, neg_cmd_gate=-10, polarity=1}
      mask prompts: f "Frequency (Hz)"; m_up "Max Input Modulation Value"; m_low "Min Input Modulation Value"; dead_time "Dead Time (s)"; pos_cmd_gate "Positive Gate Voltage (V)"; neg_cmd_gate "Negative Gate Voltage (V)"; polarity "Polarity (pu)"
  PWM generator 2 : Subsystem  mask{f=fPWM_DAB, m_up=1, m_low=0, dead_time=dead_time_DAB, pos_cmd_gate=15, neg_cmd_gate=-10, polarity=1}
      mask prompts: f "Frequency (Hz)"; m_up "Max Input Modulation Value"; m_low "Min Input Modulation Value"; dead_time "Dead Time (s)"; pos_cmd_gate "Positive Gate Voltage (V)"; neg_cmd_gate "Negative Gate Voltage (V)"; polarity "Polarity (pu)"
  PWM generator 3 : Subsystem  mask{f=fPWM_DAB, m_up=1, m_low=0, dead_time=dead_time_DAB, pos_cmd_gate=15, neg_cmd_gate=-10, polarity=1}
      mask prompts: f "Frequency (Hz)"; m_up "Max Input Modulation Value"; m_low "Min Input Modulation Value"; dead_time "Dead Time (s)"; pos_cmd_gate "Positive Gate Voltage (V)"; neg_cmd_gate "Negative Gate Voltage (V)"; polarity "Polarity (pu)"
  PWM generator 4 : Subsystem  mask{f=fPWM_DAB, m_up=1, m_low=0, dead_time=dead_time_DAB, pos_cmd_gate=15, neg_cmd_gate=-10, polarity=1}
      mask prompts: f "Frequency (Hz)"; m_up "Max Input Modulation Value"; m_low "Min Input Modulation Value"; dead_time "Dead Time (s)"; pos_cmd_gate "Positive Gate Voltage (V)"; neg_cmd_gate "Negative Gate Voltage (V)"; polarity "Polarity (pu)"
  Sum : Sum  Inputs=|++
  dab_modulation : Scope  NumInputPorts=4
      settings: SampleTime=tc  ActiveDisplayYMinimum=-13.125  ActiveDisplayYMaximum=18.125
  gate_Q1 : Outport
  gate_Q2 : Outport  Port=2
  gate_Q3 : Outport  Port=3
  gate_Q4 : Outport  Port=4
  gate_Q5 : Outport  Port=5
  gate_Q6 : Outport  Port=6
  gate_Q7 : Outport  Port=7
  gate_Q8 : Outport  Port=8
  wires:
  Constant4/1 -> Sum/2
  Constant6/1 -> PWM generator 2/2(phase)
  PWM generator 4/2(m2) -> gate_Q8/1  "gate_Q8"
  PWM generator 4/1(m1) -> gate_Q7/1, dab_modulation/4  "gate_Q7"
  PWM generator 3/2(m2) -> gate_Q6/1  "gate_Q6"
  PWM generator 3/1(m1) -> dab_modulation/3, gate_Q5/1  "gate_Q5"
  Sum/1 -> PWM generator 4/2(phase)
  Constant3/1 -> PWM generator 4/1(m_index), PWM generator 3/1(m_index)
  Gain/1 -> PWM generator 3/2(phase), Sum/1
  Constant5/1 -> PWM generator 4/3(polarity_input), PWM generator 3/3(polarity_input)
  Constant2/1 -> PWM generator 1/3(polarity_input), PWM generator 2/3(polarity_input)
  Constant1/1 -> PWM generator 1/2(phase)
  Constant/1 -> PWM generator 1/1(m_index), PWM generator 2/1(m_index)
  phase_displacement/1 -> Gain/1
  PWM generator 1/1(m1) -> dab_modulation/1, gate_Q1/1  "gate_Q1"
  PWM generator 1/2(m2) -> gate_Q2/1  "gate_Q2"
  PWM generator 2/1(m1) -> gate_Q3/1, dab_modulation/2  "gate_Q3"
  PWM generator 2/2(m2) -> gate_Q4/1  "gate_Q4"

== system sst/dab_modB/dab_ctrl/references ==
  Rate Limiter : RateLimiter  RisingSlewLimit=Vdab2_dc_nom*10  FallingSlewLimit=-Vdab2_dc_nom*10  SampleTimeMode=inherited
  Vout_dc_nom : Step  Time=1e-3  After=Vdab2_dc_nom  SampleTime=0
  vout_ref : Outport
  wires:
  Vout_dc_nom/1 -> Rate Limiter/1
  Rate Limiter/1 -> vout_ref/1

== system sst/dab_modB/dab_ctrl/sampling_i_filter1 ==
  in : Inport
  1/Ti3 : Gain  Gain=1/I_FS  OutDataTypeStr=double  SaturateOnIntegerOverflow=on  ParamDataTypeStr=Inherit: Same as input
  Unit Delay1 : UnitDelay  SampleTime=ts_dab  HasFrameUpgradeWarning=on
  Zero-Order Hold2 : ZeroOrderHold  SampleTime=ts_dab
  out_pu : Outport
  wires:
  Unit Delay1/1 -> out_pu/1
  Zero-Order Hold2/1 -> Unit Delay1/1
  1/Ti3/1 -> Zero-Order Hold2/1
  in/1 -> 1/Ti3/1

== system sst/dab_modB/dab_ctrl/sampling_v_filter1 ==
  in : Inport
  1/Ti3 : Gain  Gain=1/V_FS  OutDataTypeStr=double  SaturateOnIntegerOverflow=on  ParamDataTypeStr=Inherit: Same as input
  Unit Delay1 : UnitDelay  SampleTime=ts_dab  HasFrameUpgradeWarning=on
  Zero-Order Hold2 : ZeroOrderHold  SampleTime=ts_dab
  out_pu : Outport
  wires:
  Unit Delay1/1 -> out_pu/1
  1/Ti3/1 -> Zero-Order Hold2/1
  in/1 -> 1/Ti3/1
  Zero-Order Hold2/1 -> Unit Delay1/1

== system sst/dab_modB/dab_ctrl/sampling_v_filter2 ==
  in : Inport
  1/Ti3 : Gain  Gain=1/V_FS  OutDataTypeStr=double  SaturateOnIntegerOverflow=on  ParamDataTypeStr=Inherit: Same as input
  Saturation : Saturate  UpperLimit=1  LowerLimit=0  OutDataTypeStr=double
  Unit Delay1 : UnitDelay  SampleTime=ts_dab  HasFrameUpgradeWarning=on
  Zero-Order Hold2 : ZeroOrderHold  SampleTime=ts_dab
  out_pu : Outport
  wires:
  Unit Delay1/1 -> out_pu/1
  Saturation/1 -> Zero-Order Hold2/1
  Zero-Order Hold2/1 -> Unit Delay1/1
  1/Ti3/1 -> Saturation/1
  in/1 -> 1/Ti3/1

== system sst/dab_modB/dab_ctrl/vi ctrl ==
  i_dab_input : Inport
  u_dab_output : Inport  Port=2
  u_dab_output_ref : Inport  Port=3
  Bus Creator : BusCreator  Inputs=2
  Bus Creator1 : BusCreator  Inputs=2
  Iout Ctrl : Subsystem
  Vout Ctrl : Subsystem
  dab-tracking modB : Scope  NumInputPorts=2
      settings: ActiveDisplayYMinimum=-2  ActiveDisplayYMaximum=2  DataLoggingVariableName=ScopeData7
  u_ctrl_out_dab/i_ctrl_out_dab modB : Scope  NumInputPorts=2
      settings: ActiveDisplayYMinimum=-0.66555434270595892  ActiveDisplayYMaximum=0.14692727213509815
  phase_displacement : Outport
  tag scope: i_ctrl_out_dab_modB=global, i_in_pu_dab_modB=global, u_ctrl_out_dab_modB=global, uout_pu_dab_modB=global, uout_ref_pu_dab_modB=global
  wires:
  Bus Creator1/1 -> dab-tracking modB/2
  Bus Creator/1 -> dab-tracking modB/1
  [uout_pu_dab_modB] -> Bus Creator/2  "uout_pu_dab_modB"
  [uout_ref_pu_dab_modB] -> Bus Creator/1  "uout_ref_pu_dab_modB"
  [u_ctrl_out_dab_modB] -> Bus Creator1/1  "u_ctrl_out_dab_modB"
  [i_in_pu_dab_modB] -> Bus Creator1/2  "i_in_pu_dab_modB"
  [i_ctrl_out_dab_modB] -> u_ctrl_out_dab/i_ctrl_out_dab modB/2  "i_ctrl_out_dab"
  [u_ctrl_out_dab_modB] -> u_ctrl_out_dab/i_ctrl_out_dab modB/1  "u_ctrl_out_dab"
  Iout Ctrl/1(ctrli_out) -> phase_displacement/1, [i_ctrl_out_dab_modB]
  Vout Ctrl/1(ctrlv_out) -> [u_ctrl_out_dab_modB], Iout Ctrl/1(iout_ref)
  u_dab_output/1 -> Vout Ctrl/2(vout), [uout_pu_dab_modB]
  u_dab_output_ref/1 -> [uout_ref_pu_dab_modB], Vout Ctrl/1(vout_ref)
  i_dab_input/1 -> Iout Ctrl/2(iout), [i_in_pu_dab_modB]

== system sst/dab_modB/dc//dc with galvanic isolation/stage-1 ==
  gate_commands : Inport
  Current Sensor : fl_lib/Electrical/Electrical Sensors/Current Sensor
  PS-Simulink Converter1 : nesl_utility/PS-Simulink Converter  PhysicalDomain=network_engine_domain  SubClassName=ps_output  LeftPortType=input  RightPortType=output  PseudoPeriodic=off  Frequencies=[]  VectorFormat=1-D array  Unit=A  AffineConversion=on
  h-bridge_thermal : Subsystem  Commented=on
  h-ideal : Subsystem  Commented=on
  h-mosfet : Subsystem
  uac_1(+) : PMIOPort  Side=Left
  uac_1(-) : PMIOPort  Port=2  Side=Left
  Udc(+) : PMIOPort  Port=3  Side=Right
  Udc(-) : PMIOPort  Port=4  Side=Right
  tag scope: idc1_in_modB=global
  wires:
  PS-Simulink Converter1/1 -> [idc1_in_modB]  "idc"
  gate_commands/1 -> h-mosfet/1(gate_commands)
  connections:
  PS-Simulink Converter1/LConn1 -- Current Sensor/RConn1
  h-mosfet/RConn1 -- Current Sensor/RConn2
  Current Sensor/LConn1 -- Udc(+)/RConn1
  h-mosfet/RConn2 -- Udc(-)/RConn1
  h-mosfet/LConn2 -- uac_1(-)/RConn1
  h-mosfet/LConn1 -- uac_1(+)/RConn1

== system sst/dab_modB/dc//dc with galvanic isolation/stage-2 ==
  Current Sensor1 : fl_lib/Electrical/Electrical Sensors/Current Sensor
  PS-Simulink Converter2 : nesl_utility/PS-Simulink Converter  PhysicalDomain=network_engine_domain  SubClassName=ps_output  LeftPortType=input  RightPortType=output  PseudoPeriodic=off  Frequencies=[]  VectorFormat=1-D array  Unit=A  AffineConversion=on
  hf_trafo_center_tap_ss : Subsystem
  uac_1(+) : PMIOPort  Side=Left
  uac_2(+) : PMIOPort  Port=2  Side=Right
  uac_1(-) : PMIOPort  Port=3  Side=Left
  uac_2(-) : PMIOPort  Port=4  Side=Right
  connections:
  hf_trafo_center_tap_ss/RConn2 -- uac_2(-)/RConn1
  hf_trafo_center_tap_ss/LConn2 -- uac_1(-)/RConn1
  hf_trafo_center_tap_ss/RConn1 -- Current Sensor1/LConn1
  hf_trafo_center_tap_ss/LConn1 -- uac_1(+)/RConn1
  PS-Simulink Converter2/LConn1 -- Current Sensor1/RConn1
  Current Sensor1/RConn2 -- uac_2(+)/RConn1
